simulink model "decimate_128_test"  (R2016b)
settings: Solver=VariableStepAuto  StartTime=0.0  StopTime=2^10/Fadc  RelTol=1e-3  EnableMultiTasking=on
PreLoadFcn:
  | setup
values from neighbouring files (symbols this model uses):
  Fadc = 614.4e6    (= 614400000)    [setup.m]
libraries: xbsIndex_r4 x38, CryoDetLibCMB x1
settings Model: Creator=Mitch  LastModifiedBy=mdewart
settings OptimizationCC: LifeSpan=inf
settings DebuggingCC: SFUnexpectedBacktrackingDiag=warning  SFNoUnconditionalDefaultTransitionDiag=warning  SFExecutionAtInitializationDiag=none
settings GRTTargetCC: TargetLangStandard=C89/C90 (ANSI)  GeneratePreprocessorConditionals=Disable all
settings ConfigComp: CovMetricSettings=dw  CovHtmlReporting=on  CovSaveCumulativeToWorkspaceVar=on  CovSaveSingleToWorkspaceVar=on  CovExternalEMLEnable=off

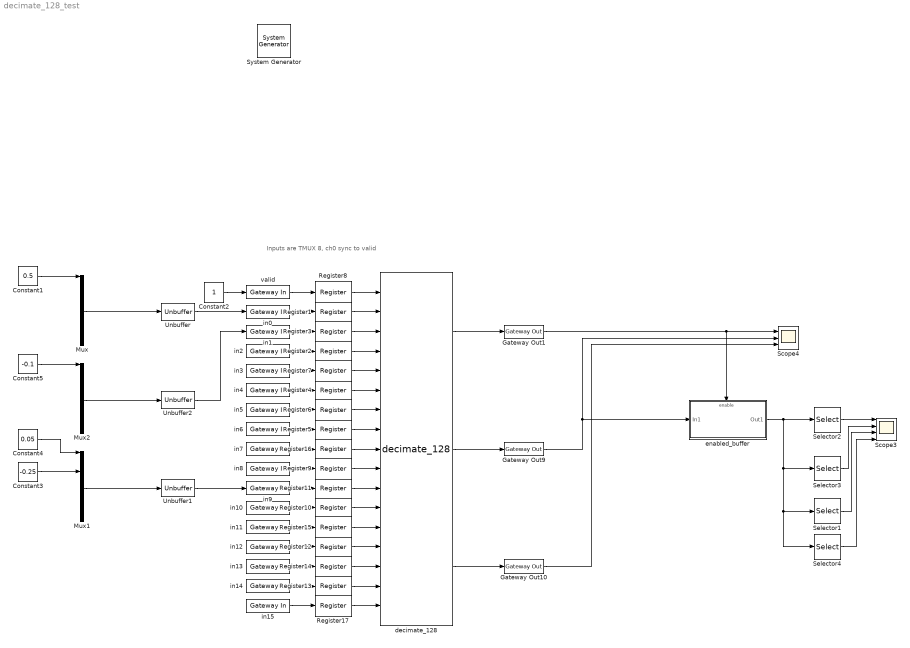
== system decimate_128_test ==
  note: Inputs are TMUX 8, ch0 sync to valid
  " System Generator" : xbsIndex_r4/ System Generator  Tag=genX  xilinxfamily=kintexu  part=xcku040  speed=-2-e  package=ffva1156  synthesis_tool=Vivado  clock_wrapper=Clock Enables  directory=./netlist  proj_type=Vivado  Synth_file=Vivado Synthesis Defaults  Impl_file=Vivado Implementation Defaults  testbench=off  simulink_period=2/Fadc  sysclk_period=2e9/Fadc  dcm_input_clock_period=10  incr_netlist=off  trim_vbits=Everywhere in SubSystem  dbl_ovrd=According to Block Masks  core_generation=According to Block Masks  run_coregen=off  deprecated_control=off  eval_field=0  block_type=sysgen
  Constant1 : Constant  Value=0.5  SampleTime=16/Fadc
  Constant2 : Constant  SampleTime=2/Fadc
  Constant3 : Constant  Value=-0.25  SampleTime=16/Fadc
  Constant4 : Constant  Value=0.05  SampleTime=16/Fadc
  Constant5 : Constant  Value=-0.1  SampleTime=16/Fadc
  Gateway Out1 : xbsIndex_r4/Gateway Out  inherit_from_input=off  hdl_port=on  rows=1  columns=1  UseAsDAC=off  DACChannel='1'  interface=None  automatic_assignment=on  address_offset=hex2dec('00')  intf_name=''  intf_description=''  timing_constraint=None  locs_specified=off  LOCs={}  io_standard={}  block_type=gatewayout
  Gateway Out10 : xbsIndex_r4/Gateway Out  inherit_from_input=off  hdl_port=on  rows=1  columns=1  UseAsDAC=off  DACChannel='1'  interface=None  automatic_assignment=on  address_offset=hex2dec('00')  intf_name=''  intf_description=''  timing_constraint=None  locs_specified=off  LOCs={}  io_standard={}  block_type=gatewayout
  Gateway Out9 : xbsIndex_r4/Gateway Out  inherit_from_input=off  hdl_port=on  rows=1  columns=1  UseAsDAC=off  DACChannel='1'  interface=None  automatic_assignment=on  address_offset=hex2dec('00')  intf_name=''  intf_description=''  timing_constraint=None  locs_specified=off  LOCs={}  io_standard={}  block_type=gatewayout
  Mux : Mux  Inputs=8
  Mux1 : Mux  Inputs=8
  Mux2 : Mux  Inputs=8
  Register{1..17} (17 alike) : xbsIndex_r4/Register  init=0  rst=off  en=off  dbl_ovrd=off  block_type=register
  Scope3 : Scope  NumInputPorts=4
  Scope4 : Scope  NumInputPorts=3
  Selector1 : Selector  InputPortWidth=128  IndexOptions=Index vector (dialog)  Indices=[9+1]  OutputSizes=1
  Selector2 : Selector  InputPortWidth=128  IndexOptions=Index vector (dialog)  Indices=[0+1]  OutputSizes=1
  Selector3 : Selector  InputPortWidth=128  IndexOptions=Index vector (dialog)  Indices=[1+1]  OutputSizes=1
  Selector4 : Selector  InputPortWidth=128  IndexOptions=Index vector (dialog)  Indices=[41+1]  OutputSizes=1
  Unbuffer : Unbuffer  SampleBasedProcessing=Same as frame based
  Unbuffer1 : Unbuffer  SampleBasedProcessing=Same as frame based
  Unbuffer2 : Unbuffer  SampleBasedProcessing=Same as frame based
  decimate_128 : CryoDetLibCMB/decimate_128
  enabled_buffer : Subsystem
  in{0..15} (16 alike) : xbsIndex_r4/Gateway In  gui_display_data_type=Fixed-point  arith_type="Signed  (2's comp)"  n_bits=18  bin_pt=15  preci_type=Single  exp_width=8  frac_width=24  rows=1  columns=1  quantization="Round  (unbiased: +/- Inf)"  overflow=Saturate  period=2/Fadc  UseAsADC=off  ADCChannel='1'  interface=None  automatic_assignment=on  address_offset=hex2dec('00')  intf_name=''  intf_description=''  default_value=0  timing_constraint=None  locs_specified=off  LOCs={}  io_standard={}  inherit_from_input=off  hdl_port=on  dbl_ovrd=off  block_type=gatewayin
  valid : xbsIndex_r4/Gateway In  gui_display_data_type=Boolean  arith_type=Boolean  n_bits=18  bin_pt=15  preci_type=Single  exp_width=8  frac_width=24  rows=1  columns=1  quantization="Round  (unbiased: +/- Inf)"  overflow=Saturate  period=2/Fadc  UseAsADC=off  ADCChannel='1'  interface=None  automatic_assignment=on  address_offset=hex2dec('00')  intf_name=''  intf_description=''  default_value=0  timing_constraint=None  locs_specified=off  LOCs={}  io_standard={}  inherit_from_input=off  hdl_port=on  dbl_ovrd=off  block_type=gatewayin
  wires:
  Constant2/1 -> valid/1
  Constant1/1 -> Mux/1
  Mux/1 -> Unbuffer/1
  Unbuffer/1 -> in0/1
  decimate_128/3 -> Gateway Out10/1
  decimate_128/1 -> Gateway Out1/1
  Gateway Out9/1 -> enabled_buffer/1(In1), Scope4/2
  Gateway Out10/1 -> Scope4/3
  Mux1/1 -> Unbuffer1/1
  Constant4/1 -> Mux1/1
  Constant3/1 -> Mux1/3
  Selector2/1 -> Scope3/1
  enabled_buffer/1(Out1) -> Selector2/1, Selector3/1, Selector4/1, Selector1/1
  Unbuffer1/1 -> in9/1
  Mux2/1 -> Unbuffer2/1
  Unbuffer2/1 -> in1/1
  Constant5/1 -> Mux2/1
  Selector3/1 -> Scope3/2
  Selector1/1 -> Scope3/3
  Selector4/1 -> Scope3/4
  in7/1 -> Register16/1
  in2/1 -> Register2/1
  in6/1 -> Register5/1
  in15/1 -> Register17/1
  valid/1 -> Register8/1
  in13/1 -> Register14/1
  in11/1 -> Register15/1
  in14/1 -> Register13/1
  in1/1 -> Register3/1
  in8/1 -> Register9/1
  in0/1 -> Register1/1
  in3/1 -> Register7/1
  in9/1 -> Register11/1
  in5/1 -> Register6/1
  in12/1 -> Register12/1
  in4/1 -> Register4/1
  in10/1 -> Register10/1
  Gateway Out1/1 -> enabled_buffer/Enable, Scope4/1
  decimate_128/2 -> Gateway Out9/1
  Register8/1 -> decimate_128/1
  Register1/1 -> decimate_128/2
  Register2/1 -> decimate_128/4
  Register3/1 -> decimate_128/3
  Register4/1 -> decimate_128/6
  Register7/1 -> decimate_128/5
  Register6/1 -> decimate_128/7
  Register5/1 -> decimate_128/8
  Register9/1 -> decimate_128/10
  Register12/1 -> decimate_128/14
  Register16/1 -> decimate_128/9
  Register13/1 -> decimate_128/16
  Register15/1 -> decimate_128/13
  Register11/1 -> decimate_128/11
  Register10/1 -> decimate_128/12
  Register14/1 -> decimate_128/15
  Register17/1 -> decimate_128/17

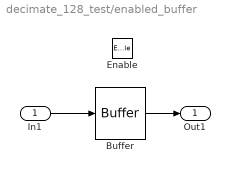
== system decimate_128_test/enabled_buffer ==
  In1 : Inport
  Enable : EnablePort
  Buffer : Buffer  N=128  TreatMby1Signals=One channel  OutputFrames=off
  Out1 : Outport
  wires:
  Buffer/1 -> Out1/1
  In1/1 -> Buffer/1
